simulink library "Butterworth"  (R2021a)
settings: Solver=VariableStepAuto  StartTime=0.0  StopTime=10.0  RelTol=1e-3
settings Model: Creator=ge26jow  LastModifiedBy=ge26jow

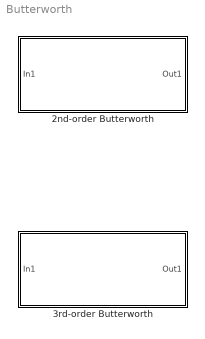
== system Butterworth ==
  2nd-order Butterworth : Subsystem  mask{Gain=1, omegac=1}
      mask prompts: Gain "DC Gain"; omegac "cuttoff frequency omega"
      mask help:
      | 2nd order Butterworth filter with input:
      | Gain and cutoff frequency
      mask Display: fprintf('2nd-order Butterworth filter')
  3rd-order Butterworth : Subsystem  mask{Gain=1, omegac=1}
      mask prompts: Gain "DC Gain"; omegac "cuttoff frequency omega"
      mask help:
      | 3rd order Butterworth filter with input:
      | Gain and cutoff frequency
      mask Display: fprintf('3rd-order Butterworth filter')

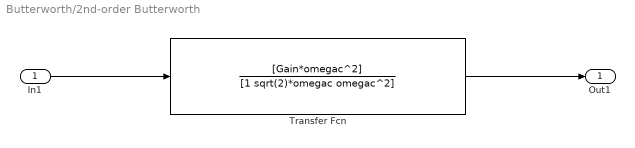
== system Butterworth/2nd-order Butterworth ==
  In1 : Inport
  Transfer Fcn : TransferFcn  Numerator=[Gain*omegac^2]  Denominator=[1 sqrt(2)*omegac omegac^2]
  Out1 : Outport
  wires:
  Transfer Fcn/1 -> Out1/1
  In1/1 -> Transfer Fcn/1

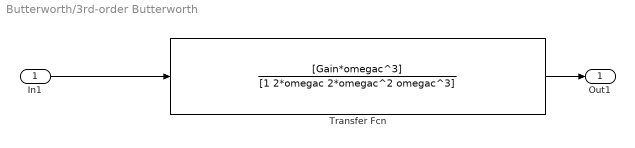
== system Butterworth/3rd-order Butterworth ==
  In1 : Inport
  Transfer Fcn : TransferFcn  Numerator=[Gain*omegac^3]  Denominator=[1 2*omegac 2*omegac^2 omegac^3]
  Out1 : Outport
  wires:
  Transfer Fcn/1 -> Out1/1
  In1/1 -> Transfer Fcn/1
